simulink model "Shuttle_Orbiter_FDM"  (R2013b)
settings: Solver=ode45  StartTime=0.0  StopTime=1000  RelTol=1e-3
values from neighbouring files (symbols this model uses):
  b = 23.79    [Orbite_InitialParamaters.m]
  c = 12.06    [Orbite_InitialParamaters.m]
  CD_alpha_mach = [0.11425	0.11975	0.13521	0.16 ... (first row only)    [Aerodynamics.m]
  CD_dbf = [0.0135	0.00959	0.0059	0.00242	-0.0005	0.00005	0.0006	0.0006 ... (first row only)    [Aerodynamics.m]
  CD_de = [0.1526	0.113	0.0796	0.0499	0.0176	-0.0262	-0.0837	-0.1391 ... (first row only)    [Aerodynamics.m]
  CDda = 0    [Aerodynamics.m]
  CDdr = 0    [Aerodynamics.m]
  CDdsb = 0.1    [Aerodynamics.m]
  CG = [1080.0 0.0 370.0]    [Orbite_InitialParamaters.m]
  CL0 = -0.05    [Aerodynamics.m]
  CL_alpha_mach = [-0.5028	-0.51097	-0.52957	-0.58454	-0.59773	-0.61005	-0.62831	-0.65514	-0.65616 ... (first row only)    [Aerodynamics.m]
  Cl_beta = [  0	0	0	0	0	0	0	0 ... (first row only)    [Aerodynamics.m]
  CLalpha = 0.05    [Aerodynamics.m]
  CLalphadot = 0    [Aerodynamics.m]
  Clbeta = -0.001    [Aerodynamics.m]
  Clda = 0.0001    [Aerodynamics.m]
  CLde = 0.02    [Aerodynamics.m]
  CLdf = 0.003    [Aerodynamics.m]
  Cldr = 0.00002    (= 2e-05)    [Aerodynamics.m]
  Cldsb = 0.000008    (= 8e-06)    [Aerodynamics.m]
  Clp = -0.003    [Aerodynamics.m]
  CLq = 0    [Aerodynamics.m]
  Clr = 0.006    [Aerodynamics.m]
  Cm0 = 0.036    [Aerodynamics.m]
  Cma = -0.012    [Aerodynamics.m]
  Cmde = -0.087    [Aerodynamics.m]
  Cmdf = -0.0017    [Aerodynamics.m]
  Cmdsb = 0.006    [Aerodynamics.m]
  Cmq = 0.058    [Aerodynamics.m]
  Cnbeta = 0.0016    [Aerodynamics.m]
  Cnda = 0.00005    (= 5e-05)    [Aerodynamics.m]
  Cndr = 0.000006    (= 6e-06)    [Aerodynamics.m]
  Cndsb = 0    [Aerodynamics.m]
  Cnp = -0.0046    [Aerodynamics.m]
  Cnr = -0.005    [Aerodynamics.m]
  CP = [1080.0 0.0 370.0]    [Orbite_InitialParamaters.m]
  CY_da = [0.00106	0.00048 	-0.00002	-0.0005     -0.0008 	-0.00102	-0.00116	-0.0014     -0.00125 ... (first row only)    [Aerodynamics.m]
  CY_de = [  -0.0004	0        0.0004	0.00096	0.0012	0.00111	0.0007	0.00045 ... (first row only)    [Aerodynamics.m]
  CY_dr = [   0.00315	0.0031	0.003	0.0029	0.00275	0.00262	0.0026	0.0026 ... (first row only)    [Aerodynamics.m]
  CY_dsb = [  0.00015 0.00007 0.00015 0.0004 0.0008	0.00133	0.002	0.0026 ... (first row only)    [Aerodynamics.m]
  CYbeta = -0.02    [Aerodynamics.m]
  CYda = 0.003    [Aerodynamics.m]
  CYdr = -0.00002    (= -2e-05)    [Aerodynamics.m]
  CYp = 0    [Aerodynamics.m]
  CYr = 0    [Aerodynamics.m]
  GlideSlopeInitial = -20    [Orbite_InitialParamaters.m]
  h_Initial = 3187+0    (= 3187)    [Orbite_InitialParamaters.m]
  heading0 = 117.5    [Orbite_InitialParamaters.m]
  HglideOrbiter = GligeSlope(:,2)    [Orbite_InitialParamaters.m]
  Iyy = 8729397    [Orbite_InitialParamaters.m]
  LongLat0 = [initial_deg(2); initial_deg(1)]    [Orbite_InitialParamaters.m]
  mass = 83000    [Orbite_InitialParamaters.m]
  runway_alt = 1    [Orbite_InitialParamaters.m]
  runway_deg = dms2degrees(runway_dms_FG)    [Orbite_InitialParamaters.m]
  S = 249.91    [Orbite_InitialParamaters.m]
  Tc = 1/25    (= 0.04)    [Orbite_InitialParamaters.m]
  XglideOrbiter = GligeSlope(:,1)    [Orbite_InitialParamaters.m]
undefined symbols (not defined in the file or in its folder): Earth, Receive, Send, WGS84
libraries: aerolibconvert2 x17, aerolibfltsims x5, simulink x3, aerolibasang x3, aerolibtransform2 x2, aerolibobsolete x1, aerolib6dof2 x1, aerolibatmos2 x1, aerolibgravity2 x1
(part 1 of 2)
settings Model: Creator=Sokol  LastModifiedBy=Sokol
settings DataIOCC: SignalLoggingSaveFormat=ModelDataLogs
settings DebuggingCC: MultiTaskDSMMsg=warning  MultiTaskCondExecSysMsg=none
settings RTWCC: IncludeERTFirstTime=on

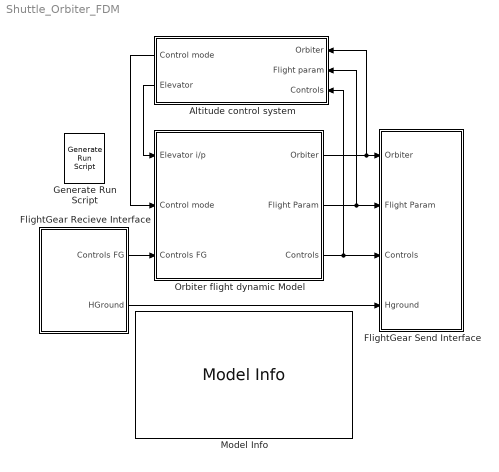
== system Shuttle_Orbiter_FDM ==
  Altitude control system : Subsystem
  FlightGear Recieve Interface : Subsystem
  FlightGear Send Interface : Subsystem
  Generate Run Script : aerolibfltsims/Generate Run Script  OutputFileName=D:\DiplomaThesis\script\runfg.bat  FlightGearBaseDirectory=C:\Program Files\FlightGear  GeometryModelName=shuttle  DestinationPort=5500  OriginAddress=127.0.0.1  OriginPort=5505  LocalAddress=127.0.0.1  AirportId=KSFO  RunwayId=10L  InitialAltitude=7224  InitialHeading=113  OffsetDistance=4.72  OffsetAzimuth=0  GenerateFile=off  Architecture=Default  dataFlow=Send-Receive
  Model Info : simulink/Model-Wide Utilities/Model Info  InitialBlockCM=None  Frame=on  DisplayStringWithTags=|  HorizontalTextAlignment=Center  LeftAlignmentValue=0.5  SourceBlockDiagram=Shuttle_Orbiter_FDM  TagMaxNumber=20
      | "Simulation Model
      | of Orbiter Flight Dynamics
      | in Langing Phase",
      | version %<ModelName>
      | Diploma Master Thesis
      | by Sokolov Alexandr
      | Politechnika Warsawska
      | June 2014,
      | %<ModifiedDate>
  Orbiter flight dynamic Model : Subsystem
      mask Display: image(imread('orbiter_pic.jpg','jpg'))
  wires:
  FlightGear Recieve Interface/2(HGround) -> FlightGear Send Interface/4(Hground)
  Orbiter flight dynamic Model/1(Orbiter) -> Altitude control system/1(Orbiter), FlightGear Send Interface/1(Orbiter)
  Orbiter flight dynamic Model/2(Flight Param) -> FlightGear Send Interface/2(Flight Param), Altitude control system/2(Flight param)
  FlightGear Recieve Interface/1(Controls FG) -> Orbiter flight dynamic Model/3(Controls FG)
  Orbiter flight dynamic Model/3(Controls) -> FlightGear Send Interface/3(Controls), Altitude control system/3(Controls)
  Altitude control system/2(Elevator) -> Orbiter flight dynamic Model/1(Elevator i/p)
  Altitude control system/1(Control mode) -> Orbiter flight dynamic Model/2(Control mode)

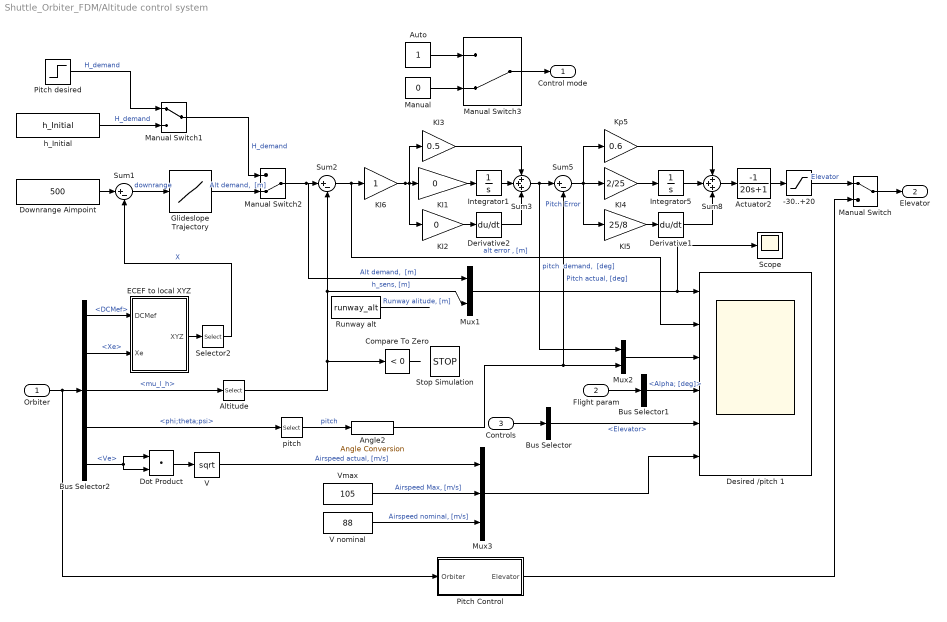
== system Shuttle_Orbiter_FDM/Altitude control system ==
  Orbiter : Inport
  Flight param : Inport  Port=2
  Controls : Inport  Port=3  SampleTime=Tc
  -30..+20 : Saturate  UpperLimit=20  LowerLimit=-35
  Actuator2 : TransferFcn  Numerator=[-1]  Denominator=[20 1]
  Altitude : Selector  InputPortWidth=3  IndexOptions=Index vector (dialog)  Indices=[3]  OutputSizes=1
  Angle2 : aerolibconvert2/Angle Conversion  IU=rad  OU=deg
  Auto : Constant
  Bus Selector : BusSelector  OutputSignals=Elevator
  Bus Selector1 : BusSelector  OutputSignals=Alpha; [deg]
  Bus Selector2 : BusSelector  OutputSignals=DCMef,Xe,mu_l_h,phi;theta;psi,Ve
  Compare To Zero : simulink/Logic and Bit Operations/Compare To Zero  relop=<  OutDataTypeStr=boolean
  Derivative1 : Derivative
  Derivative2 : Derivative
  Desired /pitch 1 : Scope  NumInputPorts=6
      settings: ShowLegends=on  YMin=1500~-40~-25~-2.5~-1~50  YMax=3250~30~15~12.5~0.75~350  SaveName=ScopeData6
  Dot Product : DotProduct  SaturateOnIntegerOverflow=on  OutDataTypeStr=Inherit: Inherit via internal rule
  Downrange Aimpoint : Constant  Value=500  OutDataTypeStr=float('double')  SampleTime=Tc
  ECEF to local XYZ : Subsystem
  Glideslope Trajectory : Lookup_n-D  NumberOfTableDimensions=1  BreakpointsForDimension1=XglideOrbiter  Table=HglideOrbiter  SaturateOnIntegerOverflow=on
  Integrator1 : Integrator
  Integrator5 : Integrator
  KI1 : Gain  Gain=0
  KI2 : Gain  Gain=0
  KI3 : Gain  Gain=0.5
  KI4 : Gain  Gain=2/25
  KI5 : Gain  Gain=25/8
  KI6 : Gain
  Kp5 : Gain  Gain=0.6
  Manual : Constant  Value=0
  Manual Switch : ManualSwitch
  Manual Switch1 : ManualSwitch
  Manual Switch2 : ManualSwitch  CurrentSetting=0
  Manual Switch3 : ManualSwitch  CurrentSetting=0
  Mux1 : Mux  Inputs=2
  Mux2 : Mux  Inputs=2
  Mux3 : Mux  Inputs=3
  Pitch Control : Subsystem
  Pitch desired : Step  Time=5  Before=h_Initial  After=h_Initial+100  SampleTime=0
  Runway alt : Constant  Value=runway_alt  OutDataTypeStr=float('double')  SampleTime=Tc
  Scope : Scope
      settings: YMin=3030  YMax=3180  SaveName=ScopeData4
  Selector2 : Selector  InputPortWidth=3  IndexOptions=Index vector (dialog)  Indices=1  OutputSizes=1
  Stop Simulation : Stop
  Sum1 : Sum  Inputs=|+-  SaturateOnIntegerOverflow=on  InputSameDT=on  OutDataTypeStr=Inherit: Same as first input
  Sum2 : Sum  Inputs=|+-  SaturateOnIntegerOverflow=on  InputSameDT=on  OutDataTypeStr=Inherit: Same as first input
  Sum3 : Sum  Inputs=+++
  Sum5 : Sum  Inputs=|+-
  Sum8 : Sum  Inputs=+++
  V : Sqrt  SaturateOnIntegerOverflow=on
  V nominal : Constant  Value=88  OutDataTypeStr=float('double')  SampleTime=Tc
  Vmax : Constant  Value=105  OutDataTypeStr=float('double')  SampleTime=Tc
  h_Initial : Constant  Value=h_Initial  OutDataTypeStr=float('double')  SampleTime=Tc
  pitch : Selector  InputPortWidth=3  IndexOptions=Index vector (dialog)  Indices=2  OutputSizes=1
  Control mode : Outport
  Elevator : Outport  Port=2
  wires:
  Bus Selector2/3 -> Altitude/1  "<mu_l_h>"
  Sum2/1 -> KI6/1, Desired /pitch 1/2  "alt error , [m]"
  Bus Selector2/4 -> pitch/1  "<phi;theta;psi>"
  pitch/1 -> Angle2/1  "pitch"
  Sum5/1 -> KI5/1, Kp5/1, KI4/1  "Pitch Error"
  Mux1/1 -> Scope/1, Desired /pitch 1/1
  Angle2/1 -> Sum5/2, Mux2/2  "Pitch actual, [deg]"
  Altitude/1 -> Compare To Zero/1, Sum2/2, Mux1/2  "h_sens, [m]"
  Bus Selector2/1 -> ECEF to local XYZ/1(DCMef)  "<DCMef>"
  Bus Selector2/2 -> ECEF to local XYZ/2(Xe)  "<Xe>"
  Downrange Aimpoint/1 -> Sum1/1
  Manual Switch2/1 -> Mux1/1, Sum2/1  "Alt demand,  [m]"
  Selector2/1 -> Sum1/2  "X"
  Sum1/1 -> Glideslope Trajectory/1  "downrange"
  -30..+20/1 -> Manual Switch/1  "Elevator"
  Bus Selector2/5 -> Dot Product/1, Dot Product/2  "<Ve>"
  Dot Product/1 -> V/1
  V/1 -> Mux3/1  "Airspeed actual, [m/s]"
  Sum8/1 -> Actuator2/1
  Orbiter/1 -> Bus Selector2/1, Pitch Control/1(Orbiter)
  Pitch Control/1(Elevator) -> Manual Switch/2
  Runway alt/1 -> ?  "Runway alitude, [m]"
  ECEF to local XYZ/1(XYZ) -> Selector2/1
  Controls/1 -> Bus Selector/1
  Bus Selector/1 -> Desired /pitch 1/5  "<Elevator>"
  Derivative1/1 -> Sum8/3
  KI5/1 -> Derivative1/1
  Integrator5/1 -> Sum8/2
  Kp5/1 -> Sum8/1
  KI4/1 -> Integrator5/1
  Compare To Zero/1 -> ?
  Flight param/1 -> Bus Selector1/1
  Bus Selector1/1 -> Desired /pitch 1/4  "<Alpha; [deg]>"
  Mux3/1 -> Desired /pitch 1/6
  Vmax/1 -> Mux3/2  "Airspeed Max, [m/s]"
  V nominal/1 -> Mux3/3  "Airspeed nominal, [m/s]"
  Manual Switch/1 -> Elevator/1
  Mux2/1 -> Desired /pitch 1/3
  Sum3/1 -> Mux2/1, Sum5/1  "pitch  demand,  [deg]"
  h_Initial/1 -> Manual Switch1/2  "H_demand"
  Pitch desired/1 -> Manual Switch1/1  "H_demand"
  Manual Switch1/1 -> Manual Switch2/1  "H_demand"
  Glideslope Trajectory/1 -> Manual Switch2/2  "Alt demand,  [m]"
  Derivative2/1 -> Sum3/3
  KI2/1 -> Derivative2/1
  Integrator1/1 -> Sum3/2
  KI3/1 -> Sum3/1
  KI1/1 -> Integrator1/1
  Actuator2/1 -> -30..+20/1
  Manual Switch3/1 -> Control mode/1
  Auto/1 -> Manual Switch3/1
  Manual/1 -> Manual Switch3/2
  KI6/1 -> KI2/1, KI3/1, KI1/1

== system Shuttle_Orbiter_FDM/FlightGear Recieve Interface ==
  note: Recieve commands from FlighGear
  note: Deflection of controls (deg):
      | Elevon: 		-35 .. +20
      | Rudder: 		+22.8
      | speed brake: 0 .. +87.2
      | body flap:  	-11.7 ... +22.5
  Bus Creator : BusCreator  Inputs=5
  Bus Creator2 : BusCreator  Inputs=5
  Bus Selector : BusSelector  OutputSignals=BodyFlap,Elevator,Aileron,Rudder,Speedbrake
  Callibration : Subsystem
  Receive net_ctrl Packet from FlightGear : aerolibfltsims/Receive net_ctrl Packet from FlightGear  FlightGearVersion=v2.10  ReceiveAddress=127.0.0.1  ReceivePort=5505  ReceiveWidth=744  varLen=off  SampleTime=1/25
      settings: AttributesFormatString=Version Selected:\n%<FlightGearVersion>
  Unpack net_ctrl Packet from FlightGear : aerolibfltsims/Unpack net_ctrl Packet from FlightGear  FlightGearVersion=v2.10  ShowControlSurfacePositionOutputs=on  ShowEngineFuelOutputs=off  ShowLandingGearOutputs=off  ShowAvionicOutputs=off  ShowEnvironmentOutputs=on  SampleTime=-1
      settings: AttributesFormatString=Version Selected: %<FlightGearVersion>
  Controls FG : Outport
  HGround : Outport  Port=2
  wires:
  Receive net_ctrl Packet from FlightGear/1 -> Unpack net_ctrl Packet from FlightGear/1
  Unpack net_ctrl Packet from FlightGear/1 -> Bus Creator/1  "Aileron"
  Unpack net_ctrl Packet from FlightGear/3 -> Bus Creator/3  "Rudder"
  Unpack net_ctrl Packet from FlightGear/7 -> Bus Creator/4  "BodyFlap"
  Unpack net_ctrl Packet from FlightGear/9 -> Bus Creator/5  "Speedbrake"
  Unpack net_ctrl Packet from FlightGear/2 -> Bus Creator/2  "Elevator"
  Bus Selector/4 -> Bus Creator2/4  "<Rudder>"
  Bus Selector/2 -> Bus Creator2/2  "<Elevator>"
  Bus Selector/3 -> Bus Creator2/3  "<Aileron>"
  Bus Selector/1 -> Bus Creator2/1  "<BodyFlap>"
  Unpack net_ctrl Packet from FlightGear/17 -> HGround/1
  Bus Selector/5 -> Bus Creator2/5  "<Speedbrake>"
  Bus Creator/1 -> Callibration/1(controns i/p)
  Bus Creator2/1 -> Controls FG/1  "AeroCon"
  Callibration/1(controls deg) -> Bus Selector/1

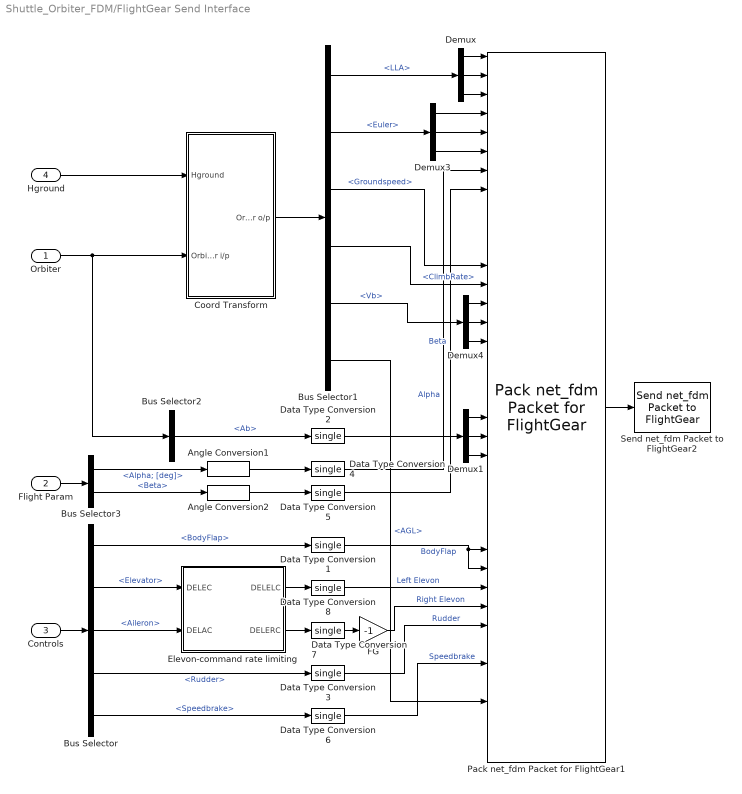
== system Shuttle_Orbiter_FDM/FlightGear Send Interface ==
  Orbiter : Inport
  Flight Param : Inport  Port=2
  Controls : Inport  Port=3
  Hground : Inport  Port=4
  Angle Conversion1 : aerolibconvert2/Angle Conversion  IU=deg  OU=rad
  Angle Conversion2 : aerolibconvert2/Angle Conversion  IU=deg  OU=rad
  Bus Selector : BusSelector  OutputSignals=BodyFlap,Elevator,Aileron,Rudder,Speedbrake
  Bus Selector1 : BusSelector  OutputSignals=LLA,Euler,Groundspeed,ClimbRate,Vb,AGL
  Bus Selector2 : BusSelector  OutputSignals=Ab
  Bus Selector3 : BusSelector  OutputSignals=Alpha; [deg],Beta
  Coord Transform : Subsystem
  Data Type Conversion{1..8} (8 alike) : DataTypeConversion  OutDataTypeStr=single
  Demux{,1,3..4} (4 alike) : Demux  Outputs=3
  Elevon-command rate limiting : Subsystem
  FG : Gain  Gain=-1
  Pack net_fdm Packet for FlightGear1 : aerolibfltsims/Pack net_fdm Packet for FlightGear  FlightGearVersion=v2.10  ShowPositionAttitudeInputs=on  ShowVelocityAccelerationInputs=on  ShowControlSurfacePositionInputs=on  ShowEngineFuelInputs=off  ShowLandingGearInputs=off  ShowEnvironmentInputs=on  SampleTime=Tc
  Send net_fdm Packet to FlightGear2 : aerolibfltsims/Send net_fdm Packet to FlightGear  DestinationIpAddress=127.0.0.1  DestinationPort=5500  LocalIpPort=-1  varLen=off  SampleTime=-1
  wires:
  Pack net_fdm Packet for FlightGear1/1 -> Send net_fdm Packet to FlightGear2/1
  Bus Selector/4 -> Data Type Conversion3/1  "<Rudder>"
  Bus Selector/1 -> Data Type Conversion1/1  "<BodyFlap>"
  Controls/1 -> Bus Selector/1
  Demux/1 -> Pack net_fdm Packet for FlightGear1/1
  Demux/2 -> Pack net_fdm Packet for FlightGear1/2
  Demux3/3 -> Pack net_fdm Packet for FlightGear1/6
  Demux3/2 -> Pack net_fdm Packet for FlightGear1/5
  Demux3/1 -> Pack net_fdm Packet for FlightGear1/4
  Orbiter/1 -> Coord Transform/2(Orbiter i/p), Bus Selector2/1
  Hground/1 -> Coord Transform/1(Hground)
  Bus Selector1/1 -> Demux/1  "<LLA>"
  Bus Selector1/2 -> Demux3/1  "<Euler>"
  Bus Selector1/3 -> Pack net_fdm Packet for FlightGear1/12  "<Groundspeed>"
  Bus Selector1/6 -> Pack net_fdm Packet for FlightGear1/35  "<AGL>"
  Bus Selector2/1 -> Data Type Conversion2/1  "<Ab>"
  Demux1/1 -> Pack net_fdm Packet for FlightGear1/20
  Demux1/2 -> Pack net_fdm Packet for FlightGear1/21
  Demux1/3 -> Pack net_fdm Packet for FlightGear1/22
  Bus Selector1/4 -> Pack net_fdm Packet for FlightGear1/13  "<ClimbRate>"
  Data Type Conversion2/1 -> Demux1/1
  Coord Transform/1(Orbiter o/p) -> Bus Selector1/1
  Demux/3 -> Pack net_fdm Packet for FlightGear1/3
  Data Type Conversion1/1 -> Pack net_fdm Packet for FlightGear1/28, Pack net_fdm Packet for FlightGear1/27  "BodyFlap"
  Data Type Conversion3/1 -> Pack net_fdm Packet for FlightGear1/31  "Rudder"
  Bus Selector/2 -> Elevon-command rate limiting/1(DELEC)  "<Elevator>"
  Bus Selector/3 -> Elevon-command rate limiting/2(DELAC)  "<Aileron>"
  Bus Selector/5 -> Data Type Conversion6/1  "<Speedbrake>"
  Data Type Conversion6/1 -> Pack net_fdm Packet for FlightGear1/33  "Speedbrake"
  Data Type Conversion7/1 -> FG/1
  Data Type Conversion8/1 -> Pack net_fdm Packet for FlightGear1/29  "Left Elevon"
  FG/1 -> Pack net_fdm Packet for FlightGear1/30  "Right Elevon"
  Elevon-command rate limiting/2(DELERC) -> Data Type Conversion7/1
  Elevon-command rate limiting/1(DELELC) -> Data Type Conversion8/1
  Flight Param/1 -> Bus Selector3/1
  Bus Selector3/1 -> Angle Conversion1/1  "<Alpha; [deg]>"
  Angle Conversion1/1 -> Data Type Conversion4/1
  Bus Selector3/2 -> Angle Conversion2/1  "<Beta>"
  Angle Conversion2/1 -> Data Type Conversion5/1
  Data Type Conversion4/1 -> Pack net_fdm Packet for FlightGear1/7  "Alpha"
  Data Type Conversion5/1 -> Pack net_fdm Packet for FlightGear1/8  "Beta"
  Demux4/1 -> Pack net_fdm Packet for FlightGear1/14
  Demux4/2 -> Pack net_fdm Packet for FlightGear1/15
  Demux4/3 -> Pack net_fdm Packet for FlightGear1/16
  Bus Selector1/5 -> Demux4/1  "<Vb>"

== system Shuttle_Orbiter_FDM/Orbiter flight dynamic Model ==
  note: Initial pos LLA (deg m)
  Elevator i/p : Inport
  Control mode : Inport  Port=2
  Controls FG : Inport  Port=3
  6DoF ECEF (Quaternion) : aerolib6dof2/6DoF ECEF (Quaternion)  units=Metric (MKS)  mtype=Fixed  xg_0="[LongLat0(2)  LongLat0(1) h_Initial]"  Vm_0=Uvw  eul_0=Euler  pm_0=pm_0  mass_0=mass  mass_e=0.5  mass_f=2.0  inertia=Inertia  inertia_e=eye(3)  inertia_f=2*eye(3)  ptype=Earth (WGS84)  F=1/298.257223563  R=6378137  w_E=7292115e-11  angle_in=Internal  LG0=0
  Aerodunamics : Subsystem
  Bus Creator2 : BusCreator  Inputs=11
  Manual / Automatic mode : Subsystem
  Total Forces & Moment : Subsystem
  Orbiter : Outport
  Flight Param : Outport  Port=2
  Controls : Outport  Port=3
  wires:
  Manual / Automatic mode/1(Controls) -> Controls/1, Aerodunamics/1(Controls)
  6DoF ECEF (Quaternion)/1 -> Bus Creator2/1  "Ve"
  6DoF ECEF (Quaternion)/2 -> Bus Creator2/2  "Xe"
  6DoF ECEF (Quaternion)/3 -> Bus Creator2/3  "mu_l_h"
  6DoF ECEF (Quaternion)/4 -> Bus Creator2/4  "phi;theta;psi"
  6DoF ECEF (Quaternion)/5 -> Bus Creator2/5  "DCM"
  6DoF ECEF (Quaternion)/6 -> Bus Creator2/6  "DCMbe"
  6DoF ECEF (Quaternion)/7 -> Bus Creator2/7  "DCMef"
  6DoF ECEF (Quaternion)/8 -> Bus Creator2/8  "Vb"
  6DoF ECEF (Quaternion)/11 -> Bus Creator2/10  "pdot_qdot_rdot"
  Bus Creator2/1 -> Total Forces & Moment/3(Orbiter), Aerodunamics/2(Orbiter), Orbiter/1
  6DoF ECEF (Quaternion)/10 -> Bus Creator2/9  "pqr"
  6DoF ECEF (Quaternion)/12 -> Bus Creator2/11  "Ab"
  Aerodunamics/2(Maero) -> Total Forces & Moment/2(Maero)
  Total Forces & Moment/2(Mcg) -> 6DoF ECEF (Quaternion)/2
  Aerodunamics/1(Faero) -> Total Forces & Moment/1(Faero)
  Aerodunamics/3(Flight Param) -> Flight Param/1
  Controls FG/1 -> Manual / Automatic mode/1(Controls FG)
  Elevator i/p/1 -> Manual / Automatic mode/2(Elevator i/p)  "Elevator"
  Total Forces & Moment/1(Fcg) -> 6DoF ECEF (Quaternion)/1
  Control mode/1 -> Manual / Automatic mode/3(Control mode)

== system Shuttle_Orbiter_FDM/Altitude control system/ECEF to local XYZ ==
  DCMef : Inport
  Xe : Inport  Port=2
  LLA to ECEF Position : aerolibtransform2/LLA to ECEF Position  units=Metric (MKS)  ptype=Earth (WGS84)  F=1/298.257223563  R=6378137
  NED to XYZ : Subsystem
  Product : Product  Multiplication=Matrix(*)  RndMeth=Zero
  "Runway altitude above MSL, m" : Constant  Value=runway_alt  SampleTime=Tc
  Runway reference coordinate (starting point) Lat Long in degrees : Constant  Value=runway_deg  SampleTime=Tc
  Sum : Sum  Inputs=|+-
  XYZ : Outport
  wires:
  Sum/1 -> Product/2
  "Runway altitude above MSL, m"/1 -> LLA to ECEF Position/2
  Runway reference coordinate (starting point) Lat Long in degrees/1 -> LLA to ECEF Position/1
  LLA to ECEF Position/1 -> Sum/2
  Product/1 -> NED to XYZ/1(NED)
  DCMef/1 -> Product/1
  NED to XYZ/1(XYZ) -> XYZ/1
  Xe/1 -> Sum/1

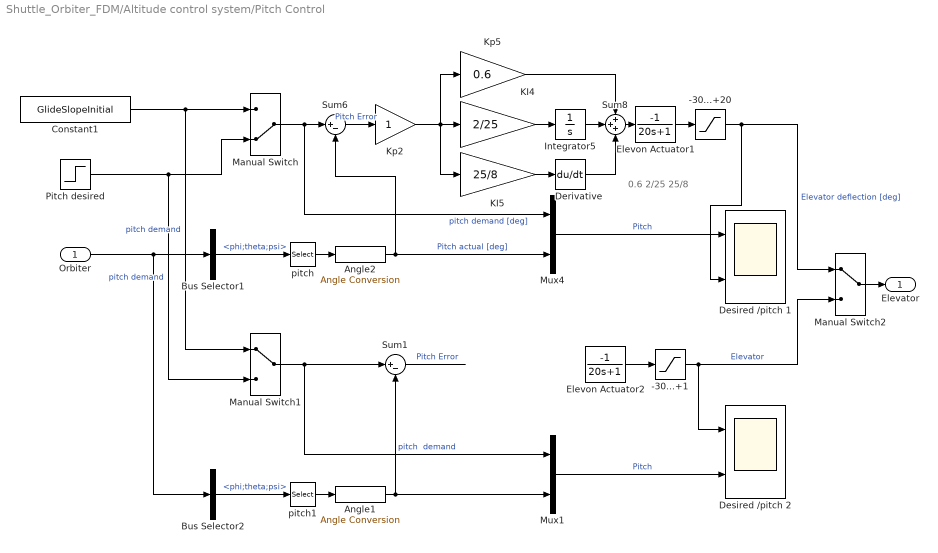
== system Shuttle_Orbiter_FDM/Altitude control system/Pitch Control ==
  note: 0.6
      | 2/25
      | 25/8
  Orbiter : Inport
  -30...+1 : Saturate  UpperLimit=20  LowerLimit=-35
  -30...+20 : Saturate  UpperLimit=20  LowerLimit=-35
  Angle1 : aerolibconvert2/Angle Conversion  IU=rad  OU=deg
  Angle2 : aerolibconvert2/Angle Conversion  IU=rad  OU=deg
  Bus Selector1 : BusSelector  OutputSignals=phi;theta;psi
  Bus Selector2 : BusSelector  OutputSignals=phi;theta;psi
  Constant1 : Constant  Value=GlideSlopeInitial
  Derivative : Derivative
  Desired /pitch 1 : Scope  NumInputPorts=2
      settings: ShowLegends=on  TimeRange=150  YMin=-20~-0.6  YMax=-13~0.05
  Desired /pitch 2 : Scope  NumInputPorts=2
      settings: YMin=-0.002~-45  YMax=0~0  SaveName=ScopeData9
  Elevon Actuator1 : TransferFcn  Numerator=[-1]  Denominator=[20 1]
  Elevon Actuator2 : TransferFcn  Numerator=[-1]  Denominator=[20 1]
  Integrator5 : Integrator
  KI4 : Gain  Gain=2/25
  KI5 : Gain  Gain=25/8
  Kp2 : Gain
  Kp5 : Gain  Gain=0.6
  Manual Switch : ManualSwitch  CurrentSetting=0
  Manual Switch1 : ManualSwitch
  Manual Switch2 : ManualSwitch
  Mux1 : Mux  Inputs=2
  Mux4 : Mux  Inputs=2
  Pitch desired : Step  Time=5  Before=GlideSlopeInitial  After=GlideSlopeInitial+5  SampleTime=0
  Sum1 : Sum  Inputs=|+-
  Sum6 : Sum  Inputs=|+-
  Sum8 : Sum  Inputs=+++
  pitch : Selector  InputPortWidth=3  IndexOptions=Index vector (dialog)  Indices=2  OutputSizes=1
  pitch1 : Selector  InputPortWidth=3  IndexOptions=Index vector (dialog)  Indices=2  OutputSizes=1
  Elevator : Outport
  wires:
  Bus Selector1/1 -> pitch/1  "<phi;theta;psi>"
  Mux4/1 -> Desired /pitch 1/1  "Pitch"
  Manual Switch/1 -> Mux4/1, Sum6/1  "pitch demand [deg]"
  pitch/1 -> Angle2/1
  -30...+20/1 -> Desired /pitch 1/2, Manual Switch2/1  "Elevator deflection [deg]"
  KI4/1 -> Integrator5/1
  Kp5/1 -> Sum8/1
  Integrator5/1 -> Sum8/2
  KI5/1 -> Derivative/1
  Derivative/1 -> Sum8/3
  Angle2/1 -> Mux4/2, Sum6/2  "Pitch actual [deg]"
  Sum6/1 -> Kp2/1  "Pitch Error"
  Bus Selector2/1 -> pitch1/1  "<phi;theta;psi>"
  Mux1/1 -> Desired /pitch 2/2  "Pitch"
  Manual Switch1/1 -> Sum1/1, Mux1/1  "pitch  demand"
  pitch1/1 -> Angle1/1
  -30...+1/1 -> Manual Switch2/2, Desired /pitch 2/1  "Elevator"
  ? -> Elevon Actuator2/1
  Angle1/1 -> Sum1/2, Mux1/2
  Orbiter/1 -> Bus Selector1/1, Bus Selector2/1
  Sum1/1 -> ?  "Pitch Error"
  Elevon Actuator2/1 -> -30...+1/1
  Constant1/1 -> Manual Switch1/1, Manual Switch/1  "pitch demand"
  Pitch desired/1 -> Manual Switch1/2, Manual Switch/2  "pitch demand"
  Manual Switch2/1 -> Elevator/1
  Kp2/1 -> Kp5/1, KI4/1, KI5/1
  Sum8/1 -> Elevon Actuator1/1
  Elevon Actuator1/1 -> -30...+20/1

== system Shuttle_Orbiter_FDM/FlightGear Recieve Interface/Callibration ==
  note: elevator and aileron is scaled to the lower range due to high sensitivity
  note: -1..+1
  note: degrees
  note: Orbiter
      | Deflection of controls (deg):
      | Elevon: 		-35 ..... +20
      | Rudder: 		-22.8....+22.8
      | speedbrake:  0.0 .... +87.2
      | body flap:  	-11.7 ... +22.5
  controns i/p : Inport
  " -11.7...+22.5" : Saturate  UpperLimit=22.5  LowerLimit=-11.7
  -22.8...+22.8 : Saturate  UpperLimit=22.8  LowerLimit=-22.8
  -35...+20 : Saturate  UpperLimit=20  LowerLimit=-35
  -35....+20 : Saturate  UpperLimit=20  LowerLimit=-35
  0...+87.2 : Saturate  UpperLimit=87.2  LowerLimit=0
  Bus Creator : BusCreator  Inputs=5
  Bus Selector : BusSelector  OutputSignals=Aileron,Elevator,Rudder,BodyFlap,Speedbrake
  Callibration coeff1 : Gain  Gain=2
  Callibration coeff2 : Gain  Gain=22.8
  Callibration coeff3 : Gain  Gain=22.5
  Callibration coeff4 : Gain  Gain=87.2
  Callibration coeff5 : Gain  Gain=2
  controls deg : Outport
  wires:
  Bus Selector/1 -> Callibration coeff5/1  "<Aileron>"
  Bus Selector/2 -> Callibration coeff1/1  "<Elevator>"
  Bus Selector/3 -> Callibration coeff2/1  "<Rudder>"
  Bus Selector/4 -> Callibration coeff3/1  "<BodyFlap>"
  Bus Selector/5 -> Callibration coeff4/1  "<Speedbrake>"
  Bus Creator/1 -> controls deg/1
  -35...+20/1 -> Bus Creator/1  "Aileron"
  -35....+20/1 -> Bus Creator/2  "Elevator"
  -22.8...+22.8/1 -> Bus Creator/3  "Rudder"
  " -11.7...+22.5"/1 -> Bus Creator/4  "BodyFlap"
  0...+87.2/1 -> Bus Creator/5  "Speedbrake"
  controns i/p/1 -> Bus Selector/1
  Callibration coeff5/1 -> -35...+20/1
  Callibration coeff1/1 -> -35....+20/1
  Callibration coeff2/1 -> -22.8...+22.8/1
  Callibration coeff3/1 -> " -11.7...+22.5"/1
  Callibration coeff4/1 -> 0...+87.2/1

== system Shuttle_Orbiter_FDM/FlightGear Send Interface/Coord Transform ==
  Hground : Inport
  Orbiter i/p : Inport  Port=2
  Angle Conversion1 : aerolibconvert2/Angle Conversion  IU=deg  OU=rad
  Angle Conversion2 : aerolibconvert2/Angle Conversion  IU=deg  OU=rad
  Angle Conversion3 : aerolibconvert2/Angle Conversion  IU=rad  OU=deg
  Angle Conversion4 : aerolibconvert2/Angle Conversion  IU=rad  OU=deg
  Angle Conversion5 : aerolibconvert2/Angle Conversion  IU=rad  OU=deg
  Bus Creator : BusCreator  Inputs=6
  Bus Selector : BusSelector  OutputSignals=phi;theta;psi,mu_l_h
  Demux2 : Demux  Outputs=3
  Demux3 : Demux  Outputs=3
  Mux5 : Mux  Inputs=2
  Mux6 : Mux  Inputs=3
  Mux9 : Mux  Inputs=3
  To Workspace1 : ToWorkspace  VariableName=Position  SampleTime=-1  SaveFormat=Timeseries
      settings: Decimation=5
  Transformations : Subsystem
  ds2 : DataTypeConversion  OutDataTypeStr=single
  Orbiter o/p : Outport
  wires:
  Orbiter i/p/1 -> Transformations/2(Plant), Bus Selector/1
  Bus Selector/2 -> Demux2/1  "<mu_l_h>"
  Bus Selector/1 -> Angle Conversion5/1, ds2/1  "<phi;theta;psi>"
  Mux5/1 -> To Workspace1/1
  Mux6/1 -> Bus Creator/6, Demux3/1  "LLA"
  Demux2/2 -> Angle Conversion2/1
  Angle Conversion1/1 -> Mux6/2
  Angle Conversion2/1 -> Mux6/1
  Demux2/3 -> Mux6/3
  Angle Conversion5/1 -> Mux5/2
  Bus Creator/1 -> Orbiter o/p/1
  Demux2/1 -> Angle Conversion1/1
  Mux9/1 -> Mux5/1
  Demux3/2 -> Angle Conversion4/1
  Angle Conversion3/1 -> Mux9/1
  Angle Conversion4/1 -> Mux9/2
  Demux3/3 -> Mux9/3
  Demux3/1 -> Angle Conversion3/1
  Hground/1 -> Transformations/1(Hground)
  Transformations/2(AGL) -> Bus Creator/2  "AGL"
  Transformations/1(Velosity) -> Bus Creator/1  "Groundspeed"
  Transformations/3(ClimbRate) -> Bus Creator/3  "ClimbRate"
  Transformations/4(Vb) -> Bus Creator/4  "Vb"
  ds2/1 -> Bus Creator/5  "Euler"

== system Shuttle_Orbiter_FDM/FlightGear Send Interface/Elevon-command rate limiting ==
  DELEC : Inport
  DELAC : Inport  Port=2
  -0.8..+0.8 : Saturate  UpperLimit=0.8  LowerLimit=-0.8
  -0.8...+0.8 : Saturate  UpperLimit=0.8  LowerLimit=-0.8
  -35..+20 : Saturate  UpperLimit=20  LowerLimit=-35
  -35...+20 : Saturate  UpperLimit=20  LowerLimit=-35
  Actuator1 : TransferFcn  Numerator=[-1]  Denominator=[20 1]
  Actuator2 : TransferFcn  Numerator=[-1]  Denominator=[20 1]
  Delay : Delay  DelayLength=1  SampleTime=Tc
  Delay1 : Delay  DelayLength=1  SampleTime=Tc
  Sum : Sum  Inputs=|+-
  Sum1 : Sum  Inputs=++|
  Sum5 : Sum  Inputs=|+-
  Sum6 : Sum  Inputs=-+|
  Sum7 : Sum  Inputs=|++
  Sum8 : Sum  Inputs=++|
  DELELC : Outport
  DELERC : Outport  Port=2
  wires:
  Delay1/1 -> Sum6/1, Sum8/1
  Sum8/1 -> Delay1/1, Actuator1/1  "DELELC"
  Delay/1 -> Sum7/2, Sum5/2
  Sum7/1 -> Delay/1, Actuator2/1  "DELERC"
  -0.8...+0.8/1 -> Sum8/2
  -0.8..+0.8/1 -> Sum7/1
  Sum6/1 -> -0.8...+0.8/1
  -35...+20/1 -> Sum6/2
  Sum5/1 -> -0.8..+0.8/1
  -35..+20/1 -> Sum5/1
  Sum1/1 -> -35...+20/1  "DELELT"
  Sum/1 -> -35..+20/1  "DELERT"
  DELAC/1 -> Sum1/2, Sum/2  "DELAC"
  DELEC/1 -> Sum/1, Sum1/1  "DELEC"
  Actuator2/1 -> DELERC/1
  Actuator1/1 -> DELELC/1

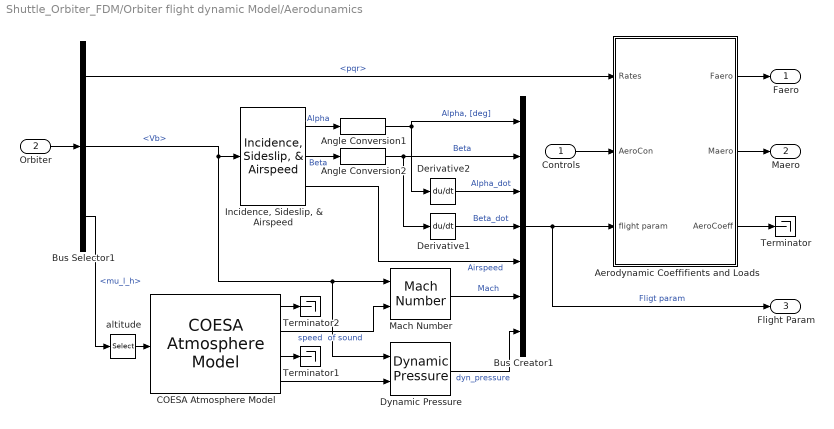
== system Shuttle_Orbiter_FDM/Orbiter flight dynamic Model/Aerodunamics ==
  Controls : Inport
  Orbiter : Inport  Port=2
  Aerodynamic Coeffifients and Loads : Subsystem
  Angle Conversion1 : aerolibconvert2/Angle Conversion  IU=rad  OU=deg
  Angle Conversion2 : aerolibconvert2/Angle Conversion  IU=rad  OU=deg
  Bus Creator1 : BusCreator  Inputs=7
  Bus Selector1 : BusSelector  OutputSignals=pqr,Vb,mu_l_h
  COESA Atmosphere Model : aerolibatmos2/COESA Atmosphere Model  units=Metric (MKS)  spec=1976 COESA-extended U.S. Standard Atmosphere  model=Profile  profile_var=High temperature  profile_percent=1%  profile_alt=5 km (16404 ft)  envelope_var=High temperature  envelope_percent=1%  action=Warning
  Derivative1 : Derivative
  Derivative2 : Derivative
  Dynamic Pressure : aerolibasang/Dynamic Pressure
  "Incidence, Sideslip, & Airspeed" : aerolibasang/Incidence, Sideslip, & Airspeed
  Mach Number : aerolibasang/Mach Number
  Terminator : Terminator
  Terminator1 : Terminator
  Terminator2 : Terminator
  altitude : Selector  InputPortWidth=3  IndexOptions=Index vector (dialog)  Indices=[3]  OutputSizes=1
  Faero : Outport
  Maero : Outport  Port=2
  Flight Param : Outport  Port=3
  wires:
  Orbiter/1 -> Bus Selector1/1
  Bus Selector1/2 -> Mach Number/1, Dynamic Pressure/1, "Incidence, Sideslip, & Airspeed"/1  "<Vb>"
  COESA Atmosphere Model/2 -> Mach Number/2  "speed  of sound"
  Angle Conversion1/1 -> Derivative2/1, Bus Creator1/1  "Alpha, [deg]"
  Bus Creator1/1 -> Aerodynamic Coeffifients and Loads/3(flight param), Flight Param/1  "Fligt param"
  "Incidence, Sideslip, & Airspeed"/2 -> Angle Conversion2/1  "Beta"
  "Incidence, Sideslip, & Airspeed"/3 -> Bus Creator1/5  "Airspeed"
  Mach Number/1 -> Bus Creator1/6  "Mach"
  COESA Atmosphere Model/4 -> Dynamic Pressure/2
  Dynamic Pressure/1 -> Bus Creator1/7  "dyn_pressure"
  Derivative2/1 -> Bus Creator1/3  "Alpha_dot"
  Derivative1/1 -> Bus Creator1/4  "Beta_dot"
  Controls/1 -> Aerodynamic Coeffifients and Loads/2(AeroCon)
  Bus Selector1/1 -> Aerodynamic Coeffifients and Loads/1(Rates)  "<pqr>"
  Aerodynamic Coeffifients and Loads/1(Faero) -> Faero/1
  Aerodynamic Coeffifients and Loads/2(Maero) -> Maero/1
  "Incidence, Sideslip, & Airspeed"/1 -> Angle Conversion1/1  "Alpha"
  Angle Conversion2/1 -> Derivative1/1, Bus Creator1/2  "Beta"
  altitude/1 -> COESA Atmosphere Model/1
  Bus Selector1/3 -> altitude/1  "<mu_l_h>"
  Aerodynamic Coeffifients and Loads/3(AeroCoeff) -> Terminator/1
  COESA Atmosphere Model/3 -> Terminator1/1
  COESA Atmosphere Model/1 -> Terminator2/1

== system Shuttle_Orbiter_FDM/Orbiter flight dynamic Model/Manual // Automatic mode ==
  Controls FG : Inport
  Elevator i/p : Inport  Port=2
  Control mode : Inport  Port=3
  Bus Creator1 : BusCreator  Inputs=5
  Bus Selector4 : BusSelector  OutputSignals=BodyFlap,Elevator,Aileron,Rudder,Speedbrake
  Switch : Switch  Criteria=u2 > Threshold
  Controls : Outport
  wires:
  Controls FG/1 -> Bus Selector4/1
  Bus Selector4/1 -> Bus Creator1/1  "<BodyFlap>"
  Bus Selector4/3 -> Bus Creator1/3  "<Aileron>"
  Bus Selector4/4 -> Bus Creator1/4  "<Rudder>"
  Switch/1 -> Bus Creator1/2  "Elevator"
  Bus Selector4/2 -> Switch/3  "<Elevator>"
  Bus Selector4/5 -> Bus Creator1/5  "<Speedbrake>"
  Bus Creator1/1 -> Controls/1
  Elevator i/p/1 -> Switch/1  "Elevator"
  Control mode/1 -> Switch/2

== system Shuttle_Orbiter_FDM/Orbiter flight dynamic Model/Total Forces & Moment ==
  note: Weight of orbiter
  note: Total Forces &  Moments
      |  at CG location
  note: Sources
  Faero : Inport  PortDimensions=[3 1]
  Maero : Inport  Port=2  PortDimensions=[3 1]
  Orbiter : Inport  Port=3
  Bus Selector1 : BusSelector  OutputSignals=mu_l_h
  Center of Gravity : Constant  Value=CG
  Center of Pressure : Constant  Value=CP
  Math Function1 : Math  Operator=transpose  SaturateOnIntegerOverflow=on
  Product : Product
  Subsystem : Subsystem
  Sum1 : Sum  Inputs=++|  SaturateOnIntegerOverflow=on  InputSameDT=on  OutDataTypeStr=Inherit: Same as first input
  Sum2 : Sum  Inputs=|+-  SaturateOnIntegerOverflow=on  InputSameDT=on  OutDataTypeStr=Inherit: Same as first input
  Sum3 : Sum  Inputs=++|  SaturateOnIntegerOverflow=on  InputSameDT=on  OutDataTypeStr=Inherit: Same as first input
  "WGS84 Gravity Model " : aerolibgravity2/WGS84 Gravity Model   model=WGS84 Taylor Series  units=Metric (MKS)  no_atmos=on  precessing=on  jd_loc=off  month=October  day=10  year=2004  no_centrifugal=on  action=Warning
  mass of orbiter : Constant  Value=mass  SampleTime=Tc
  Fcg : Outport
  Mcg : Outport  Port=2
  wires:
  Sum2/1 -> Subsystem/1(Vec1)
  Center of Gravity/1 -> Sum2/2
  Center of Pressure/1 -> Sum2/1
  Faero/1 -> Subsystem/2(Vec2), Sum3/1
  Sum1/1 -> Mcg/1
  Maero/1 -> Sum1/2
  Subsystem/1(ProdVec) -> Sum1/1
  Orbiter/1 -> Bus Selector1/1
  Bus Selector1/1 -> "WGS84 Gravity Model "/1  "<mu_l_h>"
  "WGS84 Gravity Model "/1 -> Math Function1/1
  mass of orbiter/1 -> Product/2
  Product/1 -> Sum3/2  "Weight"
  Sum3/1 -> Fcg/1
  Math Function1/1 -> Product/1

== system Shuttle_Orbiter_FDM/Altitude control system/ECEF to local XYZ/NED to XYZ ==
  NED : Inport
  Demux : Demux  Outputs=2
  E*cos : Product  RndMeth=Zero
  E*sin : Product  RndMeth=Zero
  Fcn1 : Fcn  Expr=u(1)
  Fcn2 : Fcn  Expr=u(1)
  Fcn3 : Fcn  Expr=u(1)
  Mux : Mux  Inputs=3
  N*cos : Product  RndMeth=Zero
  N*sin : Product  RndMeth=Zero
  Sel1 : Selector  InputPortWidth=3  IndexOptions=Index vector (dialog)  Indices=[1,2]  OutputSizes=1
  Sel2 : Selector  InputPortWidth=3  IndexOptions=Index vector (dialog)  Indices=3  OutputSizes=1
  SinCos : aerolibobsolete/SinCos
  Sum : Sum  Inputs=|++
  Sum1 : Sum  Inputs=|-+
  pos_deg : aerolibconvert2/Angle Conversion  IU=deg  OU=rad
  ref_pos : Constant  Value=heading0  SampleTime=Tc
  XYZ : Outport
  wires:
  Sel2/1 -> Fcn3/1
  Sel1/1 -> Demux/1
  Mux/1 -> XYZ/1
  pos_deg/1 -> SinCos/1
  Demux/2 -> E*cos/1, E*sin/1
  Sum1/1 -> Fcn2/1
  E*cos/1 -> Sum1/2
  N*sin/1 -> Sum1/1
  Sum/1 -> Fcn1/1
  E*sin/1 -> Sum/2
  SinCos/1 -> N*sin/2, E*sin/2
  N*cos/1 -> Sum/1
  SinCos/2 -> E*cos/2, N*cos/2
  Demux/1 -> N*sin/1, N*cos/1
  NED/1 -> Sel2/1, Sel1/1
  ref_pos/1 -> pos_deg/1
  Fcn1/1 -> Mux/1
  Fcn2/1 -> Mux/2
  Fcn3/1 -> Mux/3

== system Shuttle_Orbiter_FDM/FlightGear Send Interface/Coord Transform/Transformations ==
  Hground : Inport
  Plant : Inport  Port=2
  Bus Selector : BusSelector  OutputSignals=Vb,Ve,mu_l_h
  Compare To Zero : simulink/Logic and Bit Operations/Compare To Zero  relop=<  OutDataTypeStr=boolean
  Data Type Conversion : DataTypeConversion  OutDataTypeStr=single  SampleTime=Tc
  Data Type Conversion1 : DataTypeConversion  OutDataTypeStr=single
  Data Type Conversion2 : DataTypeConversion  OutDataTypeStr=single
  Data Type Conversion3 : DataTypeConversion  OutDataTypeStr=single
  Dot Product : DotProduct  SaturateOnIntegerOverflow=on  OutDataTypeStr=Inherit: Inherit via internal rule
  Integrator : Integrator
  Length Conversion : aerolibconvert2/Length Conversion  IU=m  OU=ft
  Length Conversion1 : aerolibconvert2/Length Conversion  IU=m  OU=ft
  Selector : Selector  InputPortWidth=3  IndexOptions=Index vector (dialog)  Indices=[3]  OutputSizes=1
  Stop Simulation : Stop
  Sum : Sum  Inputs=|+-
  V : Sqrt  SaturateOnIntegerOverflow=on
  Velosity : Outport
  AGL : Outport  Port=2
  ClimbRate : Outport  Port=3
  Vb : Outport  Port=4
  wires:
  Data Type Conversion3/1 -> AGL/1
  Plant/1 -> Bus Selector/1
  V/1 -> Data Type Conversion1/1
  Bus Selector/3 -> Selector/1  "<mu_l_h>"
  Bus Selector/2 -> Dot Product/1, Dot Product/2  "<Ve>"
  Dot Product/1 -> V/1
  Data Type Conversion1/1 -> Velosity/1
  Selector/1 -> Length Conversion/1, Sum/1
  Integrator/1 -> Data Type Conversion/1
  Data Type Conversion/1 -> ClimbRate/1
  Bus Selector/1 -> Length Conversion1/1  "<Vb>"
  Data Type Conversion2/1 -> Vb/1
  Hground/1 -> Sum/2
  Sum/1 -> Compare To Zero/1, Data Type Conversion3/1  "h_sens"
  Compare To Zero/1 -> Stop Simulation/1
  Length Conversion/1 -> Integrator/1
  Length Conversion1/1 -> Data Type Conversion2/1

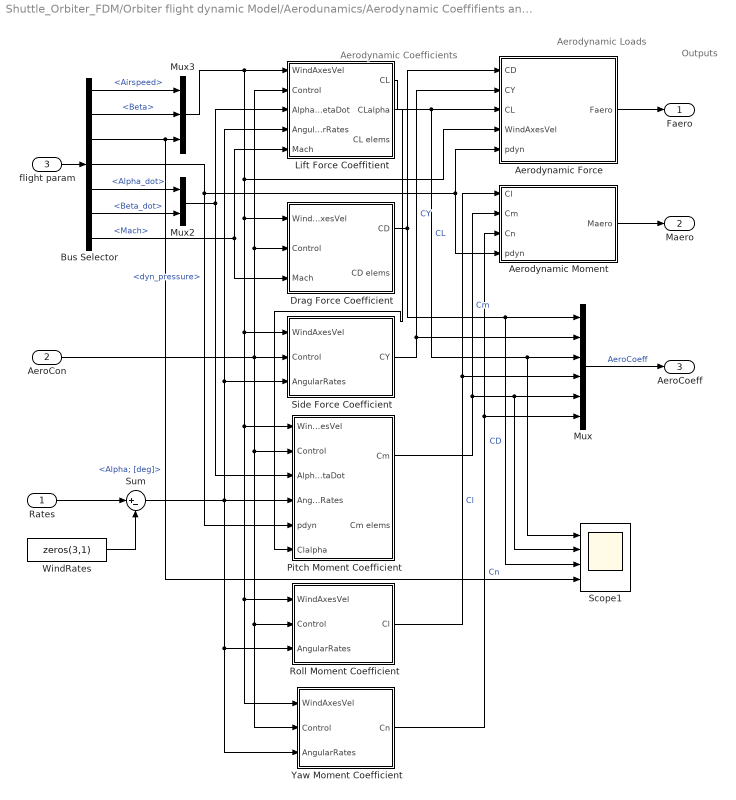
== system Shuttle_Orbiter_FDM/Orbiter flight dynamic Model/Aerodunamics/Aerodynamic Coeffifients and Loads ==
  note: Outputs
  note: Aerodynamic Coefficients
  note: Aerodynamic Loads
  Rates : Inport  PortDimensions=[3 1]
  AeroCon : Inport  Port=2
  flight param : Inport  Port=3
  Aerodynamic Force : Subsystem
  Aerodynamic Moment : Subsystem
  Bus Selector : BusSelector  OutputSignals=Airspeed,Beta,Alpha; [deg],dyn_pressure,Alpha_dot,Beta_dot,Mach
  Drag Force Coefficient : Subsystem
  Lift Force Coeffitient : Subsystem
  Mux : Mux  Inputs=6
  Mux2 : Mux  Inputs=2
  Mux3 : Mux  Inputs=3
  Pitch Moment Coefficient : Subsystem
  Roll Moment Coefficient : Subsystem
  "Scope1 " : Scope  NumInputPorts=4
      settings: ShowLegends=on  TimeRange=20  YMin=0.125~-0.015~0.06~4  YMax=0.35~0.015~0.075~8.5  SaveName=ScopeData13
  Side Force Coefficient : Subsystem
  Sum : Sum  Inputs=|+-  SaturateOnIntegerOverflow=on  InputSameDT=on  OutDataTypeStr=Inherit: Same as first input
  WindRates : Constant  Value=zeros(3,1)  SampleTime=Tc
  "Yaw Moment Coefficient " : Subsystem
  Faero : Outport
  Maero : Outport  Port=2
  AeroCoeff : Outport  Port=3
  wires:
  Sum/1 -> "Yaw Moment Coefficient "/3(AngularRates), Roll Moment Coefficient/3(AngularRates), Lift Force Coeffitient/4(AngularRates), Side Force Coefficient/3(AngularRates), Pitch Moment Coefficient/4(AngularRates)
  WindRates/1 -> Sum/2
  Rates/1 -> Sum/1
  Mux/1 -> AeroCoeff/1  "AeroCoeff"
  Aerodynamic Moment/1(Maero) -> Maero/1
  Aerodynamic Force/1(Faero) -> Faero/1
  Pitch Moment Coefficient/1(Cm) -> Aerodynamic Moment/2(Cm), "Scope1 "/2, Mux/5  "Cm"
  Roll Moment Coefficient/1(Cl) -> Mux/4, Aerodynamic Moment/1(Cl)  "Cl"
  Side Force Coefficient/1(CY) -> Mux/2, Aerodynamic Force/2(CY)  "CY"
  Drag Force Coefficient/1(CD) -> Aerodynamic Force/1(CD), "Scope1 "/3, Mux/1  "CD"
  Lift Force Coeffitient/1(CL) -> Aerodynamic Force/3(CL), "Scope1 "/1, Mux/3  "CL"
  Mux2/1 -> Lift Force Coeffitient/3(AlphaBetaDot), Pitch Moment Coefficient/3(AlphaBetaDot)
  Mux3/1 -> Side Force Coefficient/1(WindAxesVel), Pitch Moment Coefficient/1(WindAxesVel), Roll Moment Coefficient/1(WindAxesVel), "Yaw Moment Coefficient "/1(WindAxesVel), Drag Force Coefficient/1(WindAxesVel), Aerodynamic Force/4(WindAxesVel), Lift Force Coeffitient/1(WindAxesVel)
  "Yaw Moment Coefficient "/1(Cn) -> Aerodynamic Moment/3(Cn), Mux/6  "Cn"
  flight param/1 -> Bus Selector/1
  Bus Selector/2 -> Mux3/2  "<Beta>"
  Bus Selector/6 -> Mux2/2  "<Beta_dot>"
  Bus Selector/1 -> Mux3/1  "<Airspeed>"
  Bus Selector/4 -> Pitch Moment Coefficient/5(pdyn), Aerodynamic Moment/4(pdyn), Aerodynamic Force/5(pdyn)  "<dyn_pressure>"
  Bus Selector/7 -> Lift Force Coeffitient/5(Mach), Drag Force Coefficient/3(Mach)  "<Mach>"
  Bus Selector/5 -> Mux2/1  "<Alpha_dot>"
  AeroCon/1 -> Roll Moment Coefficient/2(Control), "Yaw Moment Coefficient "/2(Control), Pitch Moment Coefficient/2(Control), Lift Force Coeffitient/2(Control), Drag Force Coefficient/2(Control), Side Force Coefficient/2(Control)
  Lift Force Coeffitient/2(CLalpha) -> Pitch Moment Coefficient/6(Clalpha)
  Bus Selector/3 -> "Scope1 "/4, Mux3/3  "<Alpha; [deg]>"

== system Shuttle_Orbiter_FDM/Orbiter flight dynamic Model/Total Forces & Moment/Subsystem ==
  Vec1 : Inport
  Vec2 : Inport  Port=2
  Product : Product  SaturateOnIntegerOverflow=on  InputSameDT=on  OutDataTypeStr=Inherit: Same as first input
  Product1 : Product  SaturateOnIntegerOverflow=on  InputSameDT=on  OutDataTypeStr=Inherit: Same as first input
  Selector : Selector  InputPortWidth=3  IndexOptions=Index vector (dialog)  Indices=[2 3 1]  OutputSizes=1
  Selector1 : Selector  InputPortWidth=3  IndexOptions=Index vector (dialog)  Indices=[3 1 2]  OutputSizes=1
  Selector2 : Selector  InputPortWidth=3  IndexOptions=Index vector (dialog)  Indices=[3 1 2]  OutputSizes=1
  Selector3 : Selector  InputPortWidth=3  IndexOptions=Index vector (dialog)  Indices=[2 3 1]  OutputSizes=1
  Sum : Sum  Inputs=+-  SaturateOnIntegerOverflow=on  InputSameDT=on  OutDataTypeStr=Inherit: Same as first input
  ProdVec : Outport
  wires:
  Vec1/1 -> Selector/1, Selector2/1
  Vec2/1 -> Selector1/1, Selector3/1
  Selector/1 -> Product/1
  Selector1/1 -> Product/2
  Selector2/1 -> Product1/1
  Selector3/1 -> Product1/2
  Product/1 -> Sum/1
  Product1/1 -> Sum/2
  Sum/1 -> ProdVec/1

== system Shuttle_Orbiter_FDM/Orbiter flight dynamic Model/Aerodunamics/Aerodynamic Coeffifients and Loads/Aerodynamic Force ==
  note: Get aerodynamic forces
      | in body axes
  note: Get aerodynamic forces in
      | wind axes
  CD : Inport  PortDimensions=1
  CY : Inport  Port=2  PortDimensions=1
  CL : Inport  Port=3  PortDimensions=1
  WindAxesVel : Inport  Port=4
  pdyn : Inport  Port=5  PortDimensions=1
  Angle Conversion1 : aerolibconvert2/Angle Conversion  IU=deg  OU=rad
  Angle Conversion2 : aerolibconvert2/Angle Conversion  IU=deg  OU=rad
  ChSign : Gain  Gain=-1  SaturateOnIntegerOverflow=on  OutDataTypeStr=Inherit: Same as input  ParamDataTypeStr=Inherit: Same as input
  ChSign1 : Gain  Gain=-1  SaturateOnIntegerOverflow=on  OutDataTypeStr=Inherit: Same as input  ParamDataTypeStr=Inherit: Same as input
  DCM' : Math  Operator=transpose  SaturateOnIntegerOverflow=on
  Demux : Demux  Outputs=3
  Direction Cosine Matrix Body to Wind : aerolibtransform2/Direction Cosine Matrix Body to Wind
  Mux : Mux  Inputs=3
  Mux2 : Mux  Inputs=2
  Product : Product  Inputs=3  SaturateOnIntegerOverflow=on  InputSameDT=on  OutDataTypeStr=Inherit: Same as first input
  Product1 : Product  Multiplication=Matrix(*)  SaturateOnIntegerOverflow=on  InputSameDT=on  OutDataTypeStr=Inherit: Same as first input
  Terminator : Terminator
  Wing area : Constant  Value=S  SampleTime=0
  Faero : Outport
  wires:
  Product/1 -> Product1/2
  Direction Cosine Matrix Body to Wind/1 -> DCM'/1
  DCM'/1 -> Product1/1
  WindAxesVel/1 -> Demux/1
  Wing area/1 -> Product/3
  pdyn/1 -> Product/2
  Mux/1 -> Product/1
  CL/1 -> ChSign1/1
  CY/1 -> Mux/2
  CD/1 -> ChSign/1
  ChSign/1 -> Mux/1
  ChSign1/1 -> Mux/3
  Angle Conversion2/1 -> Mux2/1
  Angle Conversion1/1 -> Mux2/2
  Demux/3 -> Angle Conversion2/1
  Demux/2 -> Angle Conversion1/1
  Product1/1 -> Faero/1
  Mux2/1 -> Direction Cosine Matrix Body to Wind/1
  Demux/1 -> Terminator/1

== system Shuttle_Orbiter_FDM/Orbiter flight dynamic Model/Aerodunamics/Aerodynamic Coeffifients and Loads/Aerodynamic Moment ==
  note: Output
  note: Compute moments
  note: Sources
  Cl : Inport  PortDimensions=1
  Cm : Inport  Port=2  PortDimensions=1
  Cn : Inport  Port=3  PortDimensions=1
  pdyn : Inport  Port=4  PortDimensions=1
  Mux : Mux  Inputs=3
  Pitch : Product  Inputs=4  SaturateOnIntegerOverflow=on  InputSameDT=on  OutDataTypeStr=Inherit: Same as first input
  Roll : Product  Inputs=4  SaturateOnIntegerOverflow=on  InputSameDT=on  OutDataTypeStr=Inherit: Same as first input
  Wing area : Constant  Value=S
  Wing chord : Constant  Value=c
  Wing span : Constant  Value=b
  Yaw : Product  Inputs=4  SaturateOnIntegerOverflow=on  InputSameDT=on  OutDataTypeStr=Inherit: Same as first input
  Maero : Outport
  wires:
  Yaw/1 -> Mux/3
  Pitch/1 -> Mux/2
  Mux/1 -> Maero/1
  Roll/1 -> Mux/1
  Wing span/1 -> Yaw/3, Roll/3
  Wing chord/1 -> Pitch/3
  Wing area/1 -> Yaw/2, Pitch/2, Roll/2
  pdyn/1 -> Yaw/1, Pitch/1, Roll/1
  Cn/1 -> Yaw/4
  Cm/1 -> Pitch/4
  Cl/1 -> Roll/4

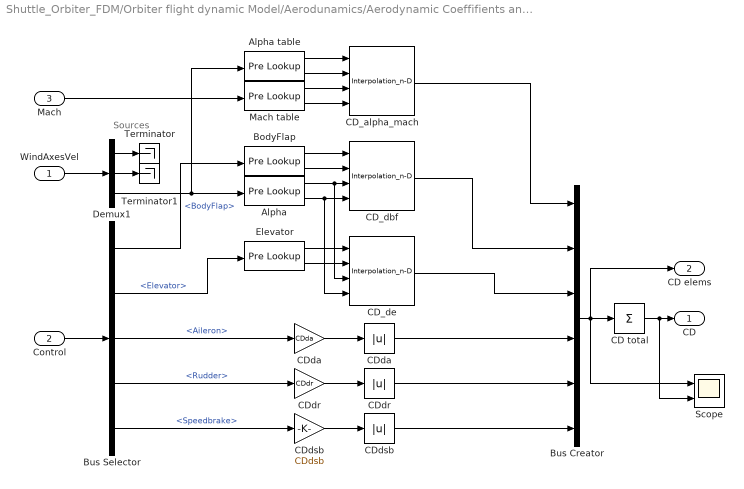
== system Shuttle_Orbiter_FDM/Orbiter flight dynamic Model/Aerodunamics/Aerodynamic Coeffifients and Loads/Drag Force Coefficient ==
  note: Sources
  WindAxesVel : Inport
  Control : Inport  Port=2
  Mach : Inport  Port=3
  Alpha : PreLookup  BreakpointsData=|  ExtrapMethod=Linear
      | [-10 -5  0	5 10 15 20 25
      | ]
  Alpha table : PreLookup  BreakpointsData=|  ExtrapMethod=Linear
      | [-10
      | -5
      | -2.5
      | 0
      | 2.5
      | 5
      | 7.5
      | 10
      | 12.5
      | 15
      | 17.5
      | 20
      | 22.5
      | 25
      | ]
  BodyFlap : PreLookup  BreakpointsData=|  ExtrapMethod=Linear
      | [-11.7
      | -5
      | 0
      | 5
      | 10
      | 16.3
      | 22.5
      | ]
  Bus Creator : BusCreator  Inputs=6
  Bus Selector : BusSelector  OutputSignals=BodyFlap,Elevator,Aileron,Rudder,Speedbrake
  CD total : Sum  Inputs=+
  CD_alpha_mach : Interpolation_n-D  Table=CD_alpha_mach  InternalRulePriority=Speed
  CD_dbf : Interpolation_n-D  Table=CD_dbf  InternalRulePriority=Speed
  CD_de : Interpolation_n-D  Table=CD_de  InternalRulePriority=Speed
  CDda : Gain  Gain=CDda  SaturateOnIntegerOverflow=on  OutDataTypeStr=Inherit: Same as input  ParamDataTypeStr=Inherit: Same as input
  "CDda " : Abs  SaturateOnIntegerOverflow=on
  CDdr : Gain  Gain=CDdr  SaturateOnIntegerOverflow=on  OutDataTypeStr=Inherit: Same as input  ParamDataTypeStr=Inherit: Same as input
  "CDdr " : Abs  SaturateOnIntegerOverflow=on
  CDdsb : Gain  Gain=CDdsb  SaturateOnIntegerOverflow=on  OutDataTypeStr=Inherit: Same as input  ParamDataTypeStr=Inherit: Same as input
  "CDdsb " : Abs  SaturateOnIntegerOverflow=on
  Demux1 : Demux  Outputs=3
  Elevator : PreLookup  BreakpointsData=|  ExtrapMethod=Linear
      | [-40
      | -35
      | -30
      | -25
      | -20
      | -15
      | -10
      | -5
      | 0
      | 5
      | 10
      | 15
      | 20
      | ]
  Mach table : PreLookup  BreakpointsData=|  ExtrapMethod=Linear
      | [0.25	0.4	0.5	0.8
      | ]
  Scope : Scope  NumInputPorts=2
      settings: ShowLegends=on  YMin=-0.01~0.07425  YMax=0.08~0.0765  SaveName=ScopeData8
  Terminator : Terminator
  Terminator1 : Terminator
  CD : Outport
  CD elems : Outport  Port=2
  wires:
  Demux1/2 -> Terminator1/1
  Demux1/1 -> Terminator/1
  "CDdr "/1 -> Bus Creator/5
  "CDda "/1 -> Bus Creator/4
  WindAxesVel/1 -> Demux1/1
  Control/1 -> Bus Selector/1
  CDda/1 -> "CDda "/1
  CDdr/1 -> "CDdr "/1
  Bus Creator/1 -> CD elems/1, Scope/1, CD total/1
  CDdsb/1 -> "CDdsb "/1
  "CDdsb "/1 -> Bus Creator/6
  Bus Selector/5 -> CDdsb/1  "<Speedbrake>"
  Bus Selector/4 -> CDdr/1  "<Rudder>"
  Bus Selector/3 -> CDda/1  "<Aileron>"
  Bus Selector/1 -> BodyFlap/1  "<BodyFlap>"
  Demux1/3 -> Alpha table/1, Alpha/1
  Elevator/1 -> CD_de/1
  Elevator/2 -> CD_de/2
  Bus Selector/2 -> Elevator/1  "<Elevator>"
  CD_de/1 -> Bus Creator/3
  Alpha/1 -> CD_de/3, CD_dbf/3
  BodyFlap/1 -> CD_dbf/1
  BodyFlap/2 -> CD_dbf/2
  Alpha/2 -> CD_de/4, CD_dbf/4
  CD_dbf/1 -> Bus Creator/2
  Mach table/1 -> CD_alpha_mach/3
  Alpha table/1 -> CD_alpha_mach/1
  Alpha table/2 -> CD_alpha_mach/2
  CD_alpha_mach/1 -> Bus Creator/1
  Mach table/2 -> CD_alpha_mach/4
  Mach/1 -> Mach table/1
  CD total/1 -> Scope/2, CD/1

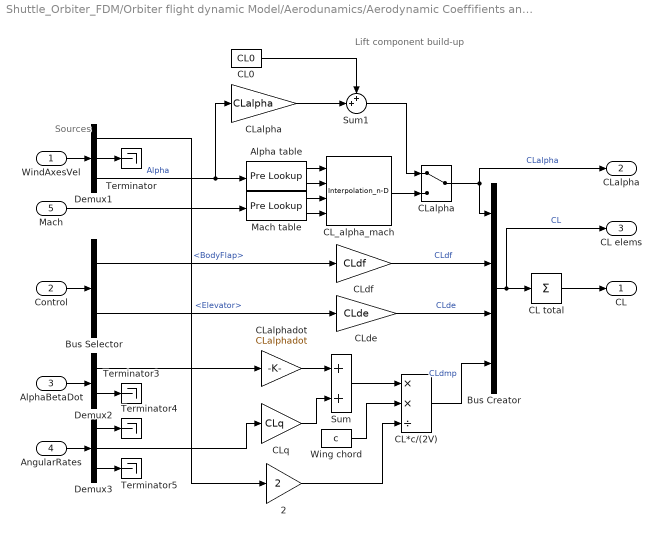
== system Shuttle_Orbiter_FDM/Orbiter flight dynamic Model/Aerodunamics/Aerodynamic Coeffifients and Loads/Lift Force Coeffitient ==
  note: Sources
  note: Lift component build-up
  WindAxesVel : Inport
  Control : Inport  Port=2
  AlphaBetaDot : Inport  Port=3
  AngularRates : Inport  Port=4
  Mach : Inport  Port=5
  2 : Gain  Gain=2  SaturateOnIntegerOverflow=on  OutDataTypeStr=Inherit: Same as input  ParamDataTypeStr=Inherit: Same as input
  Alpha table : PreLookup  BreakpointsData=|  ExtrapMethod=Linear
      | [-10
      | -5
      | -2.5
      | 0
      | 2.5
      | 5
      | 7.5
      | 10
      | 12.5
      | 15
      | 17.5
      | 20
      | 22.5
      | 25
      | ]
  Bus Creator : BusCreator
  Bus Selector : BusSelector  OutputSignals=BodyFlap,Elevator
  CL total : Sum  Inputs=+
  CL*c/(2V) : Product  Inputs=**/  SaturateOnIntegerOverflow=on  InputSameDT=on  OutDataTypeStr=Inherit: Same as first input
  CL0 : Constant  Value=CL0  SampleTime=Tc
  CL_alpha_mach : Interpolation_n-D  Table=CL_alpha_mach  InternalRulePriority=Speed
  "CLalpha " : Gain  Gain=CLalpha  SaturateOnIntegerOverflow=on  OutDataTypeStr=Inherit: Same as input  ParamDataTypeStr=Inherit: Same as input
  "CLalpha   " : ManualSwitch
  CLalphadot : Gain  Gain=CLalphadot  SaturateOnIntegerOverflow=on  OutDataTypeStr=Inherit: Same as input  ParamDataTypeStr=Inherit: Same as input
  CLde : Gain  Gain=CLde  SaturateOnIntegerOverflow=on  OutDataTypeStr=Inherit: Same as input  ParamDataTypeStr=Inherit: Same as input
  CLdf : Gain  Gain=CLdf  SaturateOnIntegerOverflow=on  OutDataTypeStr=Inherit: Same as input  ParamDataTypeStr=Inherit: Same as input
  CLq : Gain  Gain=CLq  SaturateOnIntegerOverflow=on  OutDataTypeStr=Inherit: Same as input  ParamDataTypeStr=Inherit: Same as input
  Demux1 : Demux  Outputs=3
  Demux2 : Demux  Outputs=2
  Demux3 : Demux  Outputs=3
  Mach table : PreLookup  BreakpointsData=|  ExtrapMethod=Linear
      | [0.25 0.4 0.5 0.8 0.85 0.9 0.92 0.95 0.96
      | ]
  Sum : Sum  SaturateOnIntegerOverflow=on  InputSameDT=on  OutDataTypeStr=Inherit: Same as first input
  Sum1 : Sum  Inputs=++|  SaturateOnIntegerOverflow=on  InputSameDT=on  OutDataTypeStr=Inherit: Same as first input
  Terminator{,3..5} (4 alike) : Terminator
  Wing chord : Constant  Value=c  SampleTime=Tc
  CL : Outport
  CLalpha : Outport  Port=2
  CL elems : Outport  Port=3
  wires:
  Wing chord/1 -> CL*c/(2V)/2
  CLq/1 -> Sum/2
  Demux1/1 -> 2/1
  Demux1/2 -> Terminator/1
  Control/1 -> Bus Selector/1
  Demux2/2 -> Terminator3/1
  AlphaBetaDot/1 -> Demux2/1
  CLalphadot/1 -> Sum/1
  Sum/1 -> CL*c/(2V)/1
  CLdf/1 -> Bus Creator/2  "CLdf"
  CLde/1 -> Bus Creator/3  "CLde"
  CL*c/(2V)/1 -> Bus Creator/4  "CLdmp"
  Bus Creator/1 -> CL elems/1, CL total/1  "CL"
  AngularRates/1 -> Demux3/1
  Demux3/1 -> Terminator4/1
  Demux3/2 -> CLq/1
  Demux3/3 -> Terminator5/1
  WindAxesVel/1 -> Demux1/1
  2/1 -> CL*c/(2V)/3
  Bus Selector/1 -> CLdf/1  "<BodyFlap>"
  Bus Selector/2 -> CLde/1  "<Elevator>"
  Mach table/1 -> CL_alpha_mach/3
  Alpha table/1 -> CL_alpha_mach/1
  Alpha table/2 -> CL_alpha_mach/2
  CL_alpha_mach/1 -> "CLalpha   "/2
  Mach table/2 -> CL_alpha_mach/4
  Mach/1 -> Mach table/1
  CL total/1 -> CL/1
  "CLalpha "/1 -> Sum1/2
  CL0/1 -> Sum1/1
  Sum1/1 -> "CLalpha   "/1
  "CLalpha   "/1 -> CLalpha/1, Bus Creator/1  "CLalpha"
  Demux1/3 -> "CLalpha "/1, Alpha table/1  "Alpha"
  Demux2/1 -> CLalphadot/1
